simulink model "ROPOD_4Wheel_TdistZMPC_cntr"  (R2017b)
settings: Solver=FixedStepAuto  StartTime=0.0  StopTime=Inf  FixedStep=Ts  RelTol=1e-3
PreLoadFcn:
  | cd /home/robocup/RoPod/Force_dist_ZMPC_ROS
  | init_model
InitFcn:
  | cd /home/robocup/RoPod/Force_dist_ZMPC_ROS
  | init_model
values from neighbouring files (symbols this model uses):
  b_cx = 36.5    [RoPod_parameters.mat]
  b_cy = 36.5    [RoPod_parameters.mat]
  Fd_max = 70    [RoPod_parameters.mat]
  Fd_min = 20    [RoPod_parameters.mat]
  FFtheta_intia = 0    [init_model.m]
  FFxy_mass = 80    [init_model.m]
  Fr_max = 100    [RoPod_parameters.mat]
  Fr_min = -100    [RoPod_parameters.mat]
  k_cx = 1713    [RoPod_parameters.mat]
  k_cy = 4489    [RoPod_parameters.mat]
  max_hw_tau = 7.0    (= 7)    [init_model.m]
  Nwheels = 4    [init_model.m]
  pivot_offs_sws = [2.21 1.873 2.001 3.508]    [init_model.m]
  SW_COM1_ENABLE1 = hex2dec('0001')    [init_model.m]
  SW_COM1_ENABLE2 = hex2dec('0002')    [init_model.m]
  SW_COM1_MODE_TORQUE = bitshift(hex2dec('0000'),2)    [init_model.m]
  SW_COM1_MODE_VELOCITY = bitshift(hex2dec('0002'),2)    [init_model.m]
  SW_COM1_USE_TS = hex2dec('8000')    [init_model.m]
  sw_tau_2_curr = 1/motor_physical_parameters.torqueconstant.value    [init_model.m]
  Taucompfactor = 2.0    (= 2)    [init_model.m]
  Tinit = 1*Tslot    [init_model.m]
  Ts = 0.001    [init_model.m]
  Ts_MPC = 0.001    [init_model.m]
  Tsp = 1    [init_model.m]
  xA = [1 -1 0 0 0 0 0.0206696424966 -0.0206696424966 0 0 0.0298227588181 -0.0298227588181 ... (4080 elements, 102x40)]    [ZMPCx_parameters.mat]
  xBd_dis = [1.12932348493e-06 0.000225071897401 0 0]    [ZMPCx_parameters.mat]
  xF = [0 0 0 0 0 0 0 0 0 0 0 0 ... (80 elements, 20x4)]    [ZMPCx_parameters.mat]
  xH = [20 0 0 0 0 0 0 0 0 0 0 0 ... (1600 elements, 40x40)]    [ZMPCx_parameters.mat]
  xPhi = [0.995143909015 -0.967809158823 0 0 0.980727027327 -1.91066813489 0 0 0.957042868744 -2.81984596436 0 0 ... (320 elements, 80x4)]    [ZMPCx_parameters.mat]
  xrho = 144000    [ZMPCx_parameters.mat]
  xW = [0 0 -4300 4300 0 0 -4211.12053726 4211.12053726 0 0 -4082.88267435 4082.88267435 ... (328 elements, 82x4)]    [ZMPCx_parameters.mat]
  yA = [1 -1 0 0 0 0 0.0146537039222 -0.0146537039222 0 0 0.0255124036215 -0.0255124036215 ... (4080 elements, 102x40)]    [ZMPCy_parameters.mat]
  yBd_dis = [1.24492522358e-06 0.000248362591603 0 0]    [ZMPCy_parameters.mat]
  yF = [0.00191047141222 0.00156448969707 0.00119761396088 0.000813779538874 0.00041715000072 1.20724055612e-05 -0.00039696993291 -0.000805406662726 -0.00120863105559 -0.00160205155743 -0.00198114365531 -0.00234150147928 ... (80 elements, 20x4)]    [ZMPCy_parameters.mat]
  yH = [2.00000002801 0 2.31602594113e-08 0 1.80085634996e-08 0 1.26053094289e-08 0 7.00898668547e-09 0 1.2808124932e-09 0 ... (1600 elements, 40x40)]    [ZMPCy_parameters.mat]
  yPhi = [0.994411530671 -1.11489967371 0 0 0.977778317439 -2.20691845877 0 0 0.950389393786 -3.2640842851 0 0 ... (320 elements, 80x4)]    [ZMPCy_parameters.mat]
  yrho = 10000    [ZMPCy_parameters.mat]
  yW = [0 0 -4489 4489 0 0 -4423.21952309 4423.21952309 0 0 -4308.69434324 4308.69434324 ... (328 elements, 82x4)]    [ZMPCy_parameters.mat]
undefined symbols (not defined in the file or in its folder): DiscIntNeverNeededParam, Pose, ropod_kinmodel_param, Twist, Wrench
libraries: cstblocks x85, robotlib x60, simulink x41, SOEM_EtherCAT_Lib x5, robotcorelib x1
(part 3 of 6)

== system ROPOD_4Wheel_TdistZMPC_cntr/Non-ROS Ropod Controller/velocity_setpoint/Acceleration and Velocity Limits ==
  dq_setp : Inport
  base_conf : Inport  Port=2
  Bus Selector1 : BusSelector  OutputSignals=max_acc_xy,max_vel_xy
  Bus Selector2 : BusSelector  OutputSignals=max_acc_xy,max_vel_xy
  Bus Selector3 : BusSelector  OutputSignals=max_acc_theta,max_vel_theta
  Demux : Demux  Outputs=3
  Gain{,1..5} (6 alike) : Gain  Gain=-1
  Mux : Mux  Inputs=3
  Rate Limiter Dynamic : simulink/Discontinuities/Rate Limiter Dynamic
      settings: SourceProductName=Simulink
  Rate Limiter Dynamic1 : simulink/Discontinuities/Rate Limiter Dynamic
      settings: SourceProductName=Simulink
  Rate Limiter Dynamic2 : simulink/Discontinuities/Rate Limiter Dynamic
      settings: SourceProductName=Simulink
  Saturation Dynamic : simulink/Discontinuities/Saturation Dynamic  OutMin=[]  OutMax=[]  OutDataTypeStr=Inherit: Same as second input  OutDataType=fixdt(1, 16)  OutScaling=2^-10  DoSatur=off
  Saturation Dynamic1 : simulink/Discontinuities/Saturation Dynamic  OutMin=[]  OutMax=[]  OutDataTypeStr=Inherit: Same as second input  OutDataType=fixdt(1, 16)  OutScaling=2^-10  DoSatur=off
  Saturation Dynamic2 : simulink/Discontinuities/Saturation Dynamic  OutMin=[]  OutMax=[]  OutDataTypeStr=Inherit: Same as second input  OutDataType=fixdt(1, 16)  OutScaling=2^-10  DoSatur=off
  dq_loc : Outport
  wires:
  dq_setp/1 -> Demux/1
  Gain/1 -> Rate Limiter Dynamic/3
  Demux/1 -> Saturation Dynamic/2
  Gain1/1 -> Saturation Dynamic/3
  Saturation Dynamic/1 -> Rate Limiter Dynamic/2
  Demux/2 -> Saturation Dynamic1/2
  Gain3/1 -> Saturation Dynamic1/3
  Gain2/1 -> Rate Limiter Dynamic1/3
  Saturation Dynamic1/1 -> Rate Limiter Dynamic1/2
  Bus Selector2/1 -> Rate Limiter Dynamic1/1, Gain2/1  "<max_acc_xy>"
  Bus Selector2/2 -> Saturation Dynamic1/1, Gain3/1  "<max_vel_xy>"
  Bus Selector3/1 -> Rate Limiter Dynamic2/1, Gain4/1  "<max_acc_theta>"
  Saturation Dynamic2/1 -> Rate Limiter Dynamic2/2
  base_conf/1 -> Bus Selector3/1, Bus Selector2/1, Bus Selector1/1
  Demux/3 -> Saturation Dynamic2/2
  Gain5/1 -> Saturation Dynamic2/3
  Gain4/1 -> Rate Limiter Dynamic2/3
  Bus Selector3/2 -> Saturation Dynamic2/1, Gain5/1  "<max_vel_theta>"
  Mux/1 -> dq_loc/1
  Rate Limiter Dynamic/1 -> Mux/1
  Rate Limiter Dynamic1/1 -> Mux/2
  Rate Limiter Dynamic2/1 -> Mux/3
  Bus Selector1/2 -> Saturation Dynamic/1, Gain1/1  "<max_vel_xy>"
  Bus Selector1/1 -> Rate Limiter Dynamic/1, Gain/1  "<max_acc_xy>"

== system ROPOD_4Wheel_TdistZMPC_cntr/Non-ROS Ropod Controller/velocity_setpoint/Acceleration and Velocity Limits1 ==
  note: set 0 for testing
  note: if no vel commands are received after 0.5 sec, stop
  new_cmd : Inport
  dq_setp : Inport  Port=2
  Compare To Constant : simulink/Logic and Bit Operations/Compare To Constant  relop=>=  const=0.5  OutDataTypeStr=boolean
  Constant : Constant  Value=0
  Constant1 : Constant  Value=0
  Constant2 : Constant  Value=0
  Demux : Demux  Outputs=3
  Digital Clock : DigitalClock  SampleTime=Ts
  Enabled Delay : Delay  DelayLength=1  ShowEnablePort=on  SampleTime=Ts
      settings: InputPortMap=u0,e6
  Gain6 : Gain
  Mux : Mux  Inputs=3
  Subtract : Sum  Inputs=+-
  Switch : Switch  Criteria=u2 > Threshold
  Switch1 : Switch  Criteria=u2 > Threshold
  Switch2 : Switch  Criteria=u2 > Threshold
  dq_loc : Outport
  wires:
  Demux/1 -> Switch/3
  dq_setp/1 -> Demux/1
  new_cmd/1 -> Enabled Delay/2
  Digital Clock/1 -> Enabled Delay/1, Subtract/1
  Enabled Delay/1 -> Subtract/2
  Subtract/1 -> Compare To Constant/1
  Constant/1 -> Switch/1
  Constant1/1 -> Switch1/1
  Demux/2 -> Switch1/3
  Constant2/1 -> Switch2/1
  Demux/3 -> Switch2/3
  Compare To Constant/1 -> Gain6/1
  Mux/1 -> dq_loc/1
  Gain6/1 -> Switch2/2, Switch1/2, Switch/2
  Switch/1 -> Mux/1
  Switch1/1 -> Mux/2
  Switch2/1 -> Mux/3

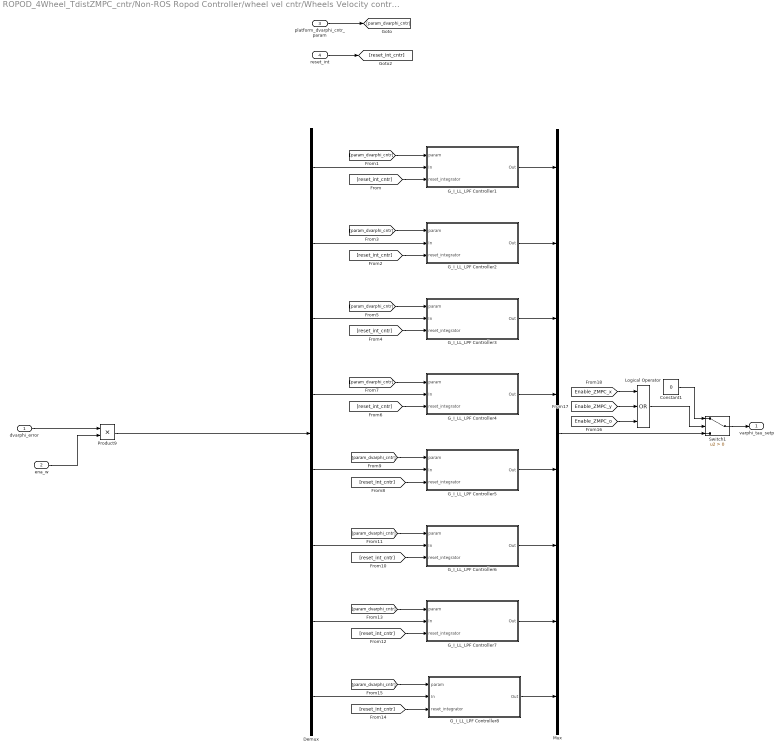
== system ROPOD_4Wheel_TdistZMPC_cntr/Non-ROS Ropod Controller/wheel vel cntr/Wheels Velocity controller ==
  dvarphi_error : Inport
  ena_w : Inport  Port=2
  platform_dvarphi_cntr_param : Inport  Port=3
  reset_int : Inport  Port=4
  Constant1 : Constant  Value=0
  Demux : Demux  Outputs=8
  G_I_LL_LPF Controller1 : Subsystem
  G_I_LL_LPF Controller2 : Subsystem
  G_I_LL_LPF Controller3 : Subsystem
  G_I_LL_LPF Controller4 : Subsystem
  G_I_LL_LPF Controller5 : Subsystem
  G_I_LL_LPF Controller6 : Subsystem
  G_I_LL_LPF Controller7 : Subsystem
  G_I_LL_LPF Controller8 : Subsystem
  Logical Operator : Logic  Operator=OR  Inputs=3  AllPortsSameDT=off  OutDataTypeStr=boolean
  Mux : Mux  Inputs=8
  Product9 : Product
  Switch1 : Switch  Criteria=u2 > Threshold
  varphi_tau_setp : Outport
  wires:
  ena_w/1 -> Product9/2
  Product9/1 -> Demux/1
  dvarphi_error/1 -> Product9/1
  [reset_int_cntr] -> G_I_LL_LPF Controller1/3(reset_integrator)
  Demux/1 -> G_I_LL_LPF Controller1/2(In)
  [param_dvarphi_cntr] -> G_I_LL_LPF Controller1/1(param)
  platform_dvarphi_cntr_param/1 -> [param_dvarphi_cntr]
  reset_int/1 -> [reset_int_cntr]
  [param_dvarphi_cntr] -> G_I_LL_LPF Controller2/1(param)
  [reset_int_cntr] -> G_I_LL_LPF Controller2/3(reset_integrator)
  Demux/2 -> G_I_LL_LPF Controller2/2(In)
  [reset_int_cntr] -> G_I_LL_LPF Controller4/3(reset_integrator)
  Demux/3 -> G_I_LL_LPF Controller3/2(In)
  Demux/4 -> G_I_LL_LPF Controller4/2(In)
  [param_dvarphi_cntr] -> G_I_LL_LPF Controller4/1(param)
  [param_dvarphi_cntr] -> G_I_LL_LPF Controller3/1(param)
  [reset_int_cntr] -> G_I_LL_LPF Controller3/3(reset_integrator)
  [param_dvarphi_cntr] -> G_I_LL_LPF Controller5/1(param)
  Demux/8 -> G_I_LL_LPF Controller8/2(In)
  [param_dvarphi_cntr] -> G_I_LL_LPF Controller7/1(param)
  [param_dvarphi_cntr] -> G_I_LL_LPF Controller8/1(param)
  [reset_int_cntr] -> G_I_LL_LPF Controller8/3(reset_integrator)
  [param_dvarphi_cntr] -> G_I_LL_LPF Controller6/1(param)
  [reset_int_cntr] -> G_I_LL_LPF Controller7/3(reset_integrator)
  Demux/6 -> G_I_LL_LPF Controller6/2(In)
  Demux/7 -> G_I_LL_LPF Controller7/2(In)
  [reset_int_cntr] -> G_I_LL_LPF Controller6/3(reset_integrator)
  [reset_int_cntr] -> G_I_LL_LPF Controller5/3(reset_integrator)
  Demux/5 -> G_I_LL_LPF Controller5/2(In)
  G_I_LL_LPF Controller1/1(Out) -> Mux/1
  G_I_LL_LPF Controller2/1(Out) -> Mux/2
  G_I_LL_LPF Controller4/1(Out) -> Mux/4
  G_I_LL_LPF Controller3/1(Out) -> Mux/3
  G_I_LL_LPF Controller5/1(Out) -> Mux/5
  G_I_LL_LPF Controller6/1(Out) -> Mux/6
  G_I_LL_LPF Controller7/1(Out) -> Mux/7
  G_I_LL_LPF Controller8/1(Out) -> Mux/8
  Constant1/1 -> Switch1/1
  Logical Operator/1 -> Switch1/2
  [Enable_ZMPC_y] -> Logical Operator/2
  [Enable_ZMPC_o] -> Logical Operator/3
  [Enable_ZMPC_x] -> Logical Operator/1
  Switch1/1 -> varphi_tau_setp/1
  Mux/1 -> Switch1/3

== system ROPOD_4Wheel_TdistZMPC_cntr/Non-ROS Ropod Controller/platform vel cntr/Bumper Interaction Controller/Angle controller ==
  angle : Inport
  Enable : EnablePort  StatesWhenEnabling=reset
  D : Gain
  Discrete-Time Integrator : DiscreteIntegrator  InitialConditionSetting=State (most efficient)  SampleTime=-1  ICPrevOutput=DiscIntNeverNeededParam  ICPrevScaledInput=DiscIntNeverNeededParam
  Discrete-Time Integrator1 : DiscreteIntegrator  InitialConditionSetting=State (most efficient)  SampleTime=-1  ICPrevOutput=DiscIntNeverNeededParam  ICPrevScaledInput=DiscIntNeverNeededParam
  I : Gain
  P : Gain  Gain=4000
  Ref_speed : Constant  Value=0
  Sum : Sum  Inputs=|+-
  Sum1 : Sum  Inputs=+|++
  Sum2 : Sum  Inputs=|+-
  u_N : Outport  OutputWhenDisabled=reset  InitialOutput=0
  wires:
  Sum1/1 -> u_N/1
  Discrete-Time Integrator/1 -> Sum1/1
  I/1 -> Discrete-Time Integrator/1
  angle/1 -> Sum2/2
  Sum2/1 -> P/1, D/1, I/1
  Ref_speed/1 -> Sum2/1
  Discrete-Time Integrator1/1 -> Sum/2
  Sum/1 -> Discrete-Time Integrator1/1, Sum1/3
  P/1 -> Sum1/2
  D/1 -> Sum/1

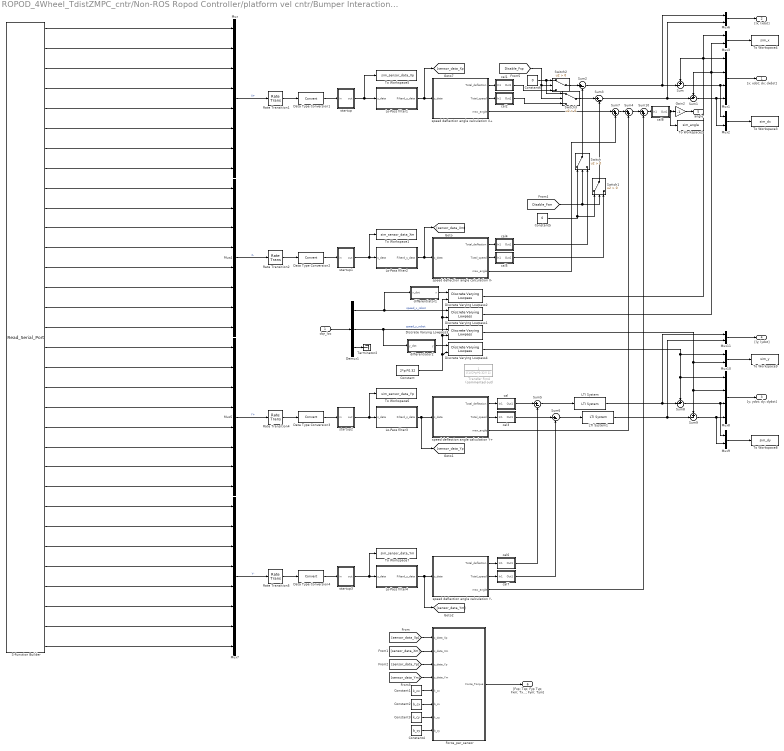
== system ROPOD_4Wheel_TdistZMPC_cntr/Non-ROS Ropod Controller/platform vel cntr/Bumper Interaction Controller/Bumper_system ==
  dqr_loc : Inport
  Constant : Constant  Value=2*pi*0.32
  Constant1 : Constant  Value=k_cx
  Constant2 : Constant  Value=b_cx
  Constant3 : Constant  Value=k_cy
  Constant4 : Constant  Value=b_cy
  Constant5 : Constant  Value=0
  Constant6 : Constant  Value=0
  Data Type Conversion{1..4} (4 alike) : DataTypeConversion
  Demux1 : Demux  Outputs=3
  Discrete Varying Lowpass{1..4} (4 alike) : cstblocks/Linear Parameter Varying/Discrete Varying Lowpass  N=1  w0=0  Ts=Ts
      settings: SourceProductName=Control System Toolbox  SourceProductBaseCode=CT
  Force_per_sensor : MATLAB Function  TreatAsAtomicUnit=on
  Gain2 : Gain  Gain=-1
  LTI System : cstblocks/LTI System  sys=hpfD_Bumper  IC=[]
  LTI System1 : cstblocks/LTI System  sys=hpfD_Bumper  IC=[]
  Lo-Pass filter1 : Subsystem
  Lo-Pass filter2 : Subsystem
  Lo-Pass filter3 : Subsystem
  Lo-Pass filter4 : Subsystem
  Mux{,4..5,7} (4 alike) : Mux  Inputs=8
  Mux1 : Mux
  Mux{2..3,6,9..11} (6 alike) : Mux  Inputs=2
  Mux8 : Mux
  Rate Transition{1..2,4..5} (4 alike) : RateTransition
  S-Function Builder : S-Function  InitFcn=try, set_param(gcb,'FunctionName','Read_Serial_Port'), end  FunctionName=Read_Serial_Port  SFunctionModules=Read_Serial_Port_wrapper  SFunctionDeploymentMode=off  EnableBusSupport=off  mask(S-Function Builder){}
      mask help: Simulink:masks:SFunctionBuilder_MD
      mask init:
      | val = [[.9  0.75 0.75 1 1 .9 .9 1]',[1 1 0.75 0.75 .9 .9 1 .9]'];try , sys = get_param(gcb,'SfunBuilderFcnName');if isempty(sys), sys = get_param(gcb,'FunctionName'); end,catch, sys = get_param(gcb,'FunctionName'); end
      settings: CopyFcn=set_param(gcbh,'LinkStatus','none')  PreSaveFcn=try, set_param(gcb,'FunctionName','Read_Serial_Port'), end  OpenFcn=sfunctionwizard(gcbh)
      mask Display: plot(val(:,1),val(:,2)),disp(sys), port_label('output',1,'dxp1'), port_label('output',2,'dxp2'), port_label('output',3,'dxp3'), port_label('output',4,'dxp4'), port_label('output',5,'sxp1'), port_label('output',6,'sxp2'), port_label('output',7,'sxp3'), port_label('output',8,'sxp4'), port_label('output',9,'dxm1'), port_label('output',10,'dxm2'), port_label('output',11,'dxm3'), port_label('output',12,'dxm4'), port_label('output',13,'sxm1'), port_label('output',14,'sxm2'), port_label('output',15,'sxm3'), port_label('output',16,'sxm4'), port_label('output',17,'dyp1'), port_label('output',18,'dyp2'), port_label('output',19,'dyp3'), port_label('output',20,'dyp4'), port_label('output',21,'syp1'), port_label('output',22,'syp2'), port_label('output',23,'syp3'), port_label('output',24,'syp4'), port_label('output',25,'dym1'), port_label('output',26,'dym2'), port_label('output',27,'dym3'), port_label('output',28,'dym4'), port_label('output',29,'sym1'), port_label('output',30,'sym2'), port_label('output',31,'sym3'), port_label('output',32,'sym4')
  Sum{,1,8..9} (4 alike) : Sum  Inputs=+-|
  Sum10 : Sum  Inputs=|++
  Sum{2..3,5..6} (4 alike) : Sum  Inputs=|+-
  Sum4 : Sum  Inputs=|++
  Sum7 : Sum  Inputs=|++
  Switch{,1..3} (4 alike) : Switch  Criteria=u2 > Threshold
  Terminator2 : Terminator
  To Workspace1 : ToWorkspace  VariableName=sim_sensor_data_Xm  SampleTime=-1
      settings: Save2DSignal=2-D array (concatenate along first dimension)
  To Workspace2 : ToWorkspace  VariableName=sim_angle  SampleTime=-1
      settings: Save2DSignal=2-D array (concatenate along first dimension)
  To Workspace3 : ToWorkspace  VariableName=sim_dx  SampleTime=-1
      settings: Save2DSignal=2-D array (concatenate along first dimension)
  To Workspace4 : ToWorkspace  VariableName=sim_x  SampleTime=-1
      settings: Save2DSignal=2-D array (concatenate along first dimension)
  To Workspace5 : ToWorkspace  VariableName=sim_sensor_data_Xp  SampleTime=-1
      settings: Save2DSignal=2-D array (concatenate along first dimension)
  To Workspace6 : ToWorkspace  VariableName=sim_sensor_data_Yp  SampleTime=-1
      settings: Save2DSignal=2-D array (concatenate along first dimension)
  To Workspace7 : ToWorkspace  VariableName=sim_sensor_data_Ym  SampleTime=-1
      settings: Save2DSignal=2-D array (concatenate along first dimension)
  To Workspace8 : ToWorkspace  VariableName=sim_dy  SampleTime=-1
      settings: Save2DSignal=2-D array (concatenate along first dimension)
  To Workspace9 : ToWorkspace  VariableName=sim_y  SampleTime=-1
      settings: Save2DSignal=2-D array (concatenate along first dimension)
  Transfer Fcn4 : TransferFcn  Commented=on  Denominator=[(1/(2*pi*0.32)) 1]
  cal : Subsystem
  cal1 : Subsystem
  cal2 : Subsystem
  cal3 : Subsystem
  cal4 : Subsystem
  cal5 : Subsystem
  cal6 : Subsystem
  cal7 : Subsystem
  cal8 : Subsystem
  differentiator1 : Subsystem
  differentiator2 : Subsystem
  speed deflection angle calculation X+ : MATLAB Function  TreatAsAtomicUnit=on
  speed deflection angle calculation X- : MATLAB Function  TreatAsAtomicUnit=on
  speed deflection angle calculation Y+ : MATLAB Function  TreatAsAtomicUnit=on
  speed deflection angle calculation Y- : MATLAB Function  TreatAsAtomicUnit=on
  startup : Subsystem
  startup1 : Subsystem
  startup2 : Subsystem
  startup3 : Subsystem
  "[x; xdot; dx; dxdot]" : Outport
  "[lx; lxdot]" : Outport  Port=2
  "[y; ydot; dy; dydot]" : Outport  Port=3
  "[ly; lydot]" : Outport  Port=4
  angle : Outport  Port=5
  "[Fxp; Txp; Fyp Typ; Fxm; Txm; Fym; Tym] " : Outport  Port=6
  wires:
  Mux2/1 -> To Workspace3/1
  Mux6/1 -> "[lx; lxdot]"/1
  Mux1/1 -> "[x; xdot; dx; dxdot]"/1
  Sum/1 -> Mux2/1, Mux1/3
  Discrete Varying Lowpass2/1 -> Mux3/1, Mux1/1, Sum/1
  Sum1/1 -> Mux2/2, Mux1/4
  Discrete Varying Lowpass1/1 -> Mux3/2, Sum1/1, Mux1/2
  Mux3/1 -> To Workspace4/1
  Demux1/3 -> Terminator2/1
  Demux1/1 -> Discrete Varying Lowpass1/1, differentiator1/1(x_dot)  "speed_x_robot"
  dqr_loc/1 -> Demux1/1
  Demux1/2 -> Discrete Varying Lowpass3/1, differentiator2/1(y_dot)  "speed_y_robot"
  differentiator1/1(x) -> Discrete Varying Lowpass2/1
  Mux/1 -> Rate Transition1/1  "X+"
  Lo-Pass filter1/1(Filterd_s_data) -> [sensor_data_Xp], speed deflection angle calculation X+/1(s_data)
  Data Type Conversion1/1 -> startup/1(in)
  Rate Transition1/1 -> Data Type Conversion1/1
  Rate Transition2/1 -> Data Type Conversion2/1
  Data Type Conversion2/1 -> startup1/1(in)
  Mux4/1 -> Rate Transition2/1  "X-"
  Rate Transition4/1 -> Data Type Conversion3/1
  Data Type Conversion3/1 -> startup2/1(in)
  Lo-Pass filter3/1(Filterd_s_data) -> [sensor_data_Yp], speed deflection angle calculation Y+/1(s_data)
  Rate Transition5/1 -> Data Type Conversion4/1
  Data Type Conversion4/1 -> startup3/1(in)
  Lo-Pass filter4/1(Filterd_s_data) -> [sensor_data_Ym], speed deflection angle calculation Y-/1(s_data)
  Mux7/1 -> Rate Transition5/1  "Y-"
  Mux5/1 -> Rate Transition4/1  "Y+"
  speed deflection angle calculation X+/1(Total_deflection) -> cal1/1(In1)
  Switch/1 -> Sum2/2
  Switch1/1 -> Sum3/2
  speed deflection angle calculation X+/3(max_angle) -> Sum7/1
  speed deflection angle calculation Y-/3(max_angle) -> Sum10/2
  speed deflection angle calculation Y-/1(Total_deflection) -> cal6/1(In1)
  speed deflection angle calculation Y+/3(max_angle) -> Sum4/2
  speed deflection angle calculation Y+/2(Total_speed) -> cal3/1(In1)
  speed deflection angle calculation Y-/2(Total_speed) -> cal7/1(In1)
  Sum8/1 -> Mux9/1, Mux8/3
  Mux10/1 -> To Workspace9/1
  Mux8/1 -> "[y; ydot; dy; dydot]"/1
  Discrete Varying Lowpass4/1 -> Mux8/1, Sum8/1, Mux10/1
  Mux11/1 -> "[ly; lydot]"/1
  Sum9/1 -> Mux9/2, Mux8/4
  Mux9/1 -> To Workspace8/1
  Discrete Varying Lowpass3/1 -> Mux8/2, Sum9/1, Mux10/2
  differentiator2/1(y) -> Discrete Varying Lowpass4/1
  speed deflection angle calculation X-/3(max_angle) -> Sum7/2
  Sum7/1 -> Sum4/1
  Sum4/1 -> Sum10/1
  Sum10/1 -> cal8/1(In1)
  Sum5/1 -> LTI System/1
  Sum2/1 -> Sum/2, Mux6/1
  Sum3/1 -> Sum1/2, Mux6/2
  Sum6/1 -> LTI System1/1
  startup/1(out) -> To Workspace5/1, Lo-Pass filter1/1(s_data)
  startup1/1(out) -> Lo-Pass filter2/1(s_data), To Workspace1/1
  startup2/1(out) -> Lo-Pass filter3/1(s_data), To Workspace6/1
  startup3/1(out) -> Lo-Pass filter4/1(s_data), To Workspace7/1
  Constant/1 -> Discrete Varying Lowpass4/2, Discrete Varying Lowpass3/2, Discrete Varying Lowpass1/2, Discrete Varying Lowpass2/2
  S-Function Builder/26 -> Mux7/2
  S-Function Builder/31 -> Mux7/7
  S-Function Builder/20 -> Mux5/4
  S-Function Builder/18 -> Mux5/2
  S-Function Builder/25 -> Mux7/1
  S-Function Builder/13 -> Mux4/5
  S-Function Builder/23 -> Mux5/7
  S-Function Builder/15 -> Mux4/7
  S-Function Builder/22 -> Mux5/6
  S-Function Builder/14 -> Mux4/6
  S-Function Builder/17 -> Mux5/1
  S-Function Builder/32 -> Mux7/8
  S-Function Builder/7 -> Mux/7
  S-Function Builder/19 -> Mux5/3
  S-Function Builder/21 -> Mux5/5
  S-Function Builder/8 -> Mux/8
  S-Function Builder/5 -> Mux/5
  S-Function Builder/4 -> Mux/4
  S-Function Builder/29 -> Mux7/5
  S-Function Builder/6 -> Mux/6
  S-Function Builder/1 -> Mux/1
  S-Function Builder/3 -> Mux/3
  S-Function Builder/10 -> Mux4/2
  S-Function Builder/11 -> Mux4/3
  S-Function Builder/12 -> Mux4/4
  S-Function Builder/16 -> Mux4/8
  S-Function Builder/28 -> Mux7/4
  S-Function Builder/27 -> Mux7/3
  S-Function Builder/9 -> Mux4/1
  S-Function Builder/30 -> Mux7/6
  S-Function Builder/2 -> Mux/2
  S-Function Builder/24 -> Mux5/8
  [sensor_data_Xp] -> Force_per_sensor/1(s_data_Xp)
  [sensor_data_Xm] -> Force_per_sensor/2(s_data_Xm)
  [sensor_data_Yp] -> Force_per_sensor/3(s_data_Yp)
  [sensor_data_Ym] -> Force_per_sensor/4(s_data_Ym)
  Force_per_sensor/1(Force_Torque) -> "[Fxp; Txp; Fyp Typ; Fxm; Txm; Fym; Tym] "/1
  Constant1/1 -> Force_per_sensor/5(k_cx)
  Constant2/1 -> Force_per_sensor/6(b_cx)
  Constant3/1 -> Force_per_sensor/7(k_cy)
  Constant4/1 -> Force_per_sensor/8(b_cy)
  cal1/1(Out1) -> Switch2/3
  speed deflection angle calculation X+/2(Total_speed) -> cal2/1(In1)
  cal2/1(Out1) -> Switch3/3
  speed deflection angle calculation X-/1(Total_deflection) -> cal4/1(In1)
  speed deflection angle calculation X-/2(Total_speed) -> cal5/1(In1)
  speed deflection angle calculation Y+/1(Total_deflection) -> cal/1(In1)
  cal/1(Out1) -> Sum5/1
  cal3/1(Out1) -> Sum6/1
  cal6/1(Out1) -> Sum5/2
  cal7/1(Out1) -> Sum6/2
  [Disable_Fxm] -> Switch/2, Switch1/2
  cal4/1(Out1) -> Switch/3
  cal5/1(Out1) -> Switch1/3
  Constant5/1 -> Switch1/1, Switch/1
  Switch2/1 -> Sum2/1
  Switch3/1 -> Sum3/1
  Constant6/1 -> Switch3/1, Switch2/1
  [Disable_Fxp] -> Switch2/2, Switch3/2
  LTI System/1 -> Sum8/2, Mux11/1
  LTI System1/1 -> Sum9/2, Mux11/2
  Lo-Pass filter2/1(Filterd_s_data) -> [sensor_data_Xm], speed deflection angle calculation X-/1(s_data)
  cal8/1(Out1) -> To Workspace2/1, Gain2/1
  Gain2/1 -> angle/1

== system ROPOD_4Wheel_TdistZMPC_cntr/Non-ROS Ropod Controller/platform vel cntr/Bumper Interaction Controller/ZMPC_x ==
  "[x; xdot; d; ddot]" : Inport
  Fd_min : Inport  Port=2
  Fd_max : Inport  Port=3
  Enable : EnablePort  StatesWhenEnabling=reset
  Constant1 : Constant  Value=xPhi
  Constant16 : Constant  Value=xH
  Constant2 : Constant  Value=xBd_dis
  Constant26 : Constant  Value=Fr_min
  Constant27 : Constant  Value=Fr_max
  Constant28 : Constant  Value=xF
  Constant30 : Constant  Value=xA
  Constant31 : Constant  Value=xW
  Constant32 : Constant  Value=xrho
  Delay{,1..4} (5 alike) : Delay  DelayLength=1  SampleTime=Ts_MPC
  Delay6 : Delay  DelayLength=1  InitialCondition=10  SampleTime=Ts_MPC
  To Workspace10 : ToWorkspace  VariableName=sim_x_e  SampleTime=-1
      settings: Save2DSignal=2-D array (concatenate along first dimension)
  To Workspace9 : ToWorkspace  VariableName=sim_x_uf  SampleTime=-1
      settings: Save2DSignal=2-D array (concatenate along first dimension)
  Zone MPC : MATLAB Function  TreatAsAtomicUnit=on  SystemSampleTime=Ts_MPC
  Fx : Outport  OutputWhenDisabled=reset  InitialOutput=0
  Feasability : Outport  Port=2  OutputWhenDisabled=reset  InitialOutput=0
  wires:
  Constant27/1 -> Zone MPC/4(Fr_max)
  Zone MPC/4(exitflag) -> Feasability/1, Delay1/1
  Delay/1 -> Zone MPC/15(mv_old)
  Delay4/1 -> Zone MPC/13(epsilon_old)
  Constant31/1 -> Zone MPC/10(W)
  Constant16/1 -> Zone MPC/7(H)
  Constant28/1 -> Zone MPC/8(F)
  Zone MPC/5(iA) -> Delay2/1
  Fd_max/1 -> Zone MPC/2(Fd_max)
  Constant26/1 -> Zone MPC/5(Fr_min)
  Delay3/1 -> Zone MPC/14(uf_old)
  Fd_min/1 -> Zone MPC/3(Fd_min)
  Constant1/1 -> Zone MPC/11(Phi)
  Zone MPC/6(s) -> Delay6/1
  Delay6/1 -> Zone MPC/18(s_old)
  Zone MPC/1(epsilon) -> To Workspace10/1, Delay4/1
  Zone MPC/2(u_f) -> To Workspace9/1, Delay3/1
  Constant32/1 -> Zone MPC/12(rho)
  Constant30/1 -> Zone MPC/9(A)
  Delay1/1 -> Zone MPC/16(exitflag_old)
  Delay2/1 -> Zone MPC/17(iA0)
  Constant2/1 -> Zone MPC/6(Bd_dis)
  "[x; xdot; d; ddot]"/1 -> Zone MPC/1(mo)
  Zone MPC/3(mv) -> Delay/1, Fx/1

== system ROPOD_4Wheel_TdistZMPC_cntr/Non-ROS Ropod Controller/platform vel cntr/Bumper Interaction Controller/ZMPC_y ==
  "[x; xdot; d; ddot]" : Inport
  Fd_min : Inport  Port=2
  Fd_max : Inport  Port=3
  Enable : EnablePort  StatesWhenEnabling=reset
  Constant1 : Constant  Value=yPhi
  Constant16 : Constant  Value=yH
  Constant2 : Constant  Value=yBd_dis
  Constant26 : Constant  Value=Fr_min
  Constant27 : Constant  Value=Fr_max
  Constant28 : Constant  Value=yF
  Constant30 : Constant  Value=yA
  Constant31 : Constant  Value=yW
  Constant32 : Constant  Value=yrho
  Delay{,1..4} (5 alike) : Delay  DelayLength=1  SampleTime=Ts_MPC
  Delay6 : Delay  DelayLength=1  InitialCondition=10  SampleTime=Ts_MPC
  To Workspace10 : ToWorkspace  VariableName=sim_y_e  SampleTime=-1
      settings: Save2DSignal=2-D array (concatenate along first dimension)
  To Workspace9 : ToWorkspace  VariableName=sim_y_uf  SampleTime=-1
      settings: Save2DSignal=2-D array (concatenate along first dimension)
  Zone MPC : MATLAB Function  TreatAsAtomicUnit=on  SystemSampleTime=Ts_MPC
  Fx : Outport  OutputWhenDisabled=reset  InitialOutput=0
  Feasability : Outport  Port=2  OutputWhenDisabled=reset  InitialOutput=0
  wires:
  Zone MPC/3(mv) -> Fx/1, Delay/1
  "[x; xdot; d; ddot]"/1 -> Zone MPC/1(mo)
  Constant2/1 -> Zone MPC/6(Bd_dis)
  Delay2/1 -> Zone MPC/17(iA0)
  Delay1/1 -> Zone MPC/16(exitflag_old)
  Constant30/1 -> Zone MPC/9(A)
  Constant32/1 -> Zone MPC/12(rho)
  Zone MPC/2(u_f) -> Delay3/1, To Workspace9/1
  Zone MPC/1(epsilon) -> Delay4/1, To Workspace10/1
  Delay6/1 -> Zone MPC/18(s_old)
  Zone MPC/6(s) -> Delay6/1
  Constant1/1 -> Zone MPC/11(Phi)
  Fd_min/1 -> Zone MPC/3(Fd_min)
  Delay3/1 -> Zone MPC/14(uf_old)
  Constant26/1 -> Zone MPC/5(Fr_min)
  Fd_max/1 -> Zone MPC/2(Fd_max)
  Zone MPC/5(iA) -> Delay2/1
  Constant28/1 -> Zone MPC/8(F)
  Constant16/1 -> Zone MPC/7(H)
  Constant31/1 -> Zone MPC/10(W)
  Delay4/1 -> Zone MPC/13(epsilon_old)
  Delay/1 -> Zone MPC/15(mv_old)
  Zone MPC/4(exitflag) -> Delay1/1, Feasability/1
  Constant27/1 -> Zone MPC/4(Fr_max)

== system ROPOD_4Wheel_TdistZMPC_cntr/Non-ROS Ropod Controller/platform vel cntr/Platorm Velocity controller/G_I_LL_LPF Controller1 ==
  param : Inport
  In : Inport  Port=2
  reset_integrator : Inport  Port=3
  Bus Selector : BusSelector  OutputSignals=P_gain,I_freq_hz,LL_zero_fhz,LL_pole_fhz,LPF_fhz
  Discrete Varying Lowpass3 : cstblocks/Linear Parameter Varying/Discrete Varying Lowpass  N=1  w0=0  Ts=Ts
      settings: SourceProductName=Control System Toolbox  SourceProductBaseCode=CT
  Gain2 : Gain  Gain=2*pi
  Product5 : Product
  Shapeit Integrator (Tustin) : Subsystem
  Shapeit Lead-Lag (Tustin) : Subsystem
  Out : Outport
  wires:
  Gain2/1 -> Discrete Varying Lowpass3/2
  Product5/1 -> Shapeit Integrator (Tustin)/1(In)
  Discrete Varying Lowpass3/1 -> Out/1
  Shapeit Integrator (Tustin)/1(Out) -> Shapeit Lead-Lag (Tustin)/1(In)
  Bus Selector/1 -> Product5/2  "<P_gain>"
  Bus Selector/2 -> Shapeit Integrator (Tustin)/2(I_fhz)  "<I_freq_hz>"
  param/1 -> Bus Selector/1
  Bus Selector/5 -> Gain2/1  "<LPF_fhz>"
  Bus Selector/4 -> Shapeit Lead-Lag (Tustin)/3(fp)  "<LL_pole_fhz>"
  reset_integrator/1 -> Shapeit Integrator (Tustin)/3(reset)
  Bus Selector/3 -> Shapeit Lead-Lag (Tustin)/2(fz)  "<LL_zero_fhz>"
  Shapeit Lead-Lag (Tustin)/1(Out) -> Discrete Varying Lowpass3/1
  In/1 -> Product5/1

== system ROPOD_4Wheel_TdistZMPC_cntr/Non-ROS Ropod Controller/platform vel cntr/Platorm Velocity controller/G_I_LL_LPF Controller2 ==
  param : Inport
  In : Inport  Port=2
  reset_integrator : Inport  Port=3
  Bus Selector : BusSelector  OutputSignals=P_gain,I_freq_hz,LL_zero_fhz,LL_pole_fhz,LPF_fhz
  Discrete Varying Lowpass3 : cstblocks/Linear Parameter Varying/Discrete Varying Lowpass  N=1  w0=0  Ts=Ts
      settings: SourceProductName=Control System Toolbox  SourceProductBaseCode=CT
  Gain2 : Gain  Gain=2*pi
  Product5 : Product
  Shapeit Integrator (Tustin) : Subsystem
  Shapeit Lead-Lag (Tustin) : Subsystem
  Out : Outport
  wires:
  Gain2/1 -> Discrete Varying Lowpass3/2
  Product5/1 -> Shapeit Integrator (Tustin)/1(In)
  Discrete Varying Lowpass3/1 -> Out/1
  Shapeit Integrator (Tustin)/1(Out) -> Shapeit Lead-Lag (Tustin)/1(In)
  Bus Selector/1 -> Product5/2  "<P_gain>"
  Bus Selector/2 -> Shapeit Integrator (Tustin)/2(I_fhz)  "<I_freq_hz>"
  param/1 -> Bus Selector/1
  Bus Selector/5 -> Gain2/1  "<LPF_fhz>"
  Bus Selector/4 -> Shapeit Lead-Lag (Tustin)/3(fp)  "<LL_pole_fhz>"
  reset_integrator/1 -> Shapeit Integrator (Tustin)/3(reset)
  Bus Selector/3 -> Shapeit Lead-Lag (Tustin)/2(fz)  "<LL_zero_fhz>"
  Shapeit Lead-Lag (Tustin)/1(Out) -> Discrete Varying Lowpass3/1
  In/1 -> Product5/1

== system ROPOD_4Wheel_TdistZMPC_cntr/Non-ROS Ropod Controller/platform vel cntr/Platorm Velocity controller/G_I_LL_LPF Controller3 ==
  param : Inport
  In : Inport  Port=2
  reset_integrator : Inport  Port=3
  Bus Selector : BusSelector  OutputSignals=P_gain,I_freq_hz,LL_zero_fhz,LL_pole_fhz,LPF_fhz
  Discrete Varying Lowpass3 : cstblocks/Linear Parameter Varying/Discrete Varying Lowpass  N=1  w0=0  Ts=Ts
      settings: SourceProductName=Control System Toolbox  SourceProductBaseCode=CT
  Gain2 : Gain  Gain=2*pi
  Product5 : Product
  Shapeit Integrator (Tustin) : Subsystem
  Shapeit Lead-Lag (Tustin) : Subsystem
  Out : Outport
  wires:
  Gain2/1 -> Discrete Varying Lowpass3/2
  Product5/1 -> Shapeit Integrator (Tustin)/1(In)
  Discrete Varying Lowpass3/1 -> Out/1
  Shapeit Integrator (Tustin)/1(Out) -> Shapeit Lead-Lag (Tustin)/1(In)
  Bus Selector/1 -> Product5/2  "<P_gain>"
  Bus Selector/2 -> Shapeit Integrator (Tustin)/2(I_fhz)  "<I_freq_hz>"
  param/1 -> Bus Selector/1
  Bus Selector/5 -> Gain2/1  "<LPF_fhz>"
  Bus Selector/4 -> Shapeit Lead-Lag (Tustin)/3(fp)  "<LL_pole_fhz>"
  reset_integrator/1 -> Shapeit Integrator (Tustin)/3(reset)
  Bus Selector/3 -> Shapeit Lead-Lag (Tustin)/2(fz)  "<LL_zero_fhz>"
  Shapeit Lead-Lag (Tustin)/1(Out) -> Discrete Varying Lowpass3/1
  In/1 -> Product5/1

== system ROPOD_4Wheel_TdistZMPC_cntr/Non-ROS Ropod Controller/wheel vel cntr/Wheels Velocity controller/G_I_LL_LPF Controller1 ==
  param : Inport
  In : Inport  Port=2
  reset_integrator : Inport  Port=3
  Bus Selector : BusSelector  OutputSignals=P_gain,I_freq_hz,LL_zero_fhz,LL_pole_fhz,LPF_fhz
  Discrete Varying Lowpass3 : cstblocks/Linear Parameter Varying/Discrete Varying Lowpass  N=1  w0=0  Ts=Ts
      settings: SourceProductName=Control System Toolbox  SourceProductBaseCode=CT
  Gain2 : Gain  Gain=2*pi
  Product5 : Product
  Shapeit Integrator (Tustin) : Subsystem
  Shapeit Lead-Lag (Tustin) : Subsystem
  Out : Outport
  wires:
  Gain2/1 -> Discrete Varying Lowpass3/2
  Product5/1 -> Shapeit Integrator (Tustin)/1(In)
  Discrete Varying Lowpass3/1 -> Out/1
  Shapeit Integrator (Tustin)/1(Out) -> Shapeit Lead-Lag (Tustin)/1(In)
  Bus Selector/1 -> Product5/2  "<P_gain>"
  Bus Selector/2 -> Shapeit Integrator (Tustin)/2(I_fhz)  "<I_freq_hz>"
  param/1 -> Bus Selector/1
  Bus Selector/5 -> Gain2/1  "<LPF_fhz>"
  Bus Selector/4 -> Shapeit Lead-Lag (Tustin)/3(fp)  "<LL_pole_fhz>"
  reset_integrator/1 -> Shapeit Integrator (Tustin)/3(reset)
  Bus Selector/3 -> Shapeit Lead-Lag (Tustin)/2(fz)  "<LL_zero_fhz>"
  Shapeit Lead-Lag (Tustin)/1(Out) -> Discrete Varying Lowpass3/1
  In/1 -> Product5/1

== system ROPOD_4Wheel_TdistZMPC_cntr/Non-ROS Ropod Controller/wheel vel cntr/Wheels Velocity controller/G_I_LL_LPF Controller2 ==
  param : Inport
  In : Inport  Port=2
  reset_integrator : Inport  Port=3
  Bus Selector : BusSelector  OutputSignals=P_gain,I_freq_hz,LL_zero_fhz,LL_pole_fhz,LPF_fhz
  Discrete Varying Lowpass3 : cstblocks/Linear Parameter Varying/Discrete Varying Lowpass  N=1  w0=0  Ts=Ts
      settings: SourceProductName=Control System Toolbox  SourceProductBaseCode=CT
  Gain2 : Gain  Gain=2*pi
  Product5 : Product
  Shapeit Integrator (Tustin) : Subsystem
  Shapeit Lead-Lag (Tustin) : Subsystem
  Out : Outport
  wires:
  Gain2/1 -> Discrete Varying Lowpass3/2
  Product5/1 -> Shapeit Integrator (Tustin)/1(In)
  Discrete Varying Lowpass3/1 -> Out/1
  Shapeit Integrator (Tustin)/1(Out) -> Shapeit Lead-Lag (Tustin)/1(In)
  Bus Selector/1 -> Product5/2  "<P_gain>"
  Bus Selector/2 -> Shapeit Integrator (Tustin)/2(I_fhz)  "<I_freq_hz>"
  param/1 -> Bus Selector/1
  Bus Selector/5 -> Gain2/1  "<LPF_fhz>"
  Bus Selector/4 -> Shapeit Lead-Lag (Tustin)/3(fp)  "<LL_pole_fhz>"
  reset_integrator/1 -> Shapeit Integrator (Tustin)/3(reset)
  Bus Selector/3 -> Shapeit Lead-Lag (Tustin)/2(fz)  "<LL_zero_fhz>"
  Shapeit Lead-Lag (Tustin)/1(Out) -> Discrete Varying Lowpass3/1
  In/1 -> Product5/1

== system ROPOD_4Wheel_TdistZMPC_cntr/Non-ROS Ropod Controller/wheel vel cntr/Wheels Velocity controller/G_I_LL_LPF Controller3 ==
  param : Inport
  In : Inport  Port=2
  reset_integrator : Inport  Port=3
  Bus Selector : BusSelector  OutputSignals=P_gain,I_freq_hz,LL_zero_fhz,LL_pole_fhz,LPF_fhz
  Discrete Varying Lowpass3 : cstblocks/Linear Parameter Varying/Discrete Varying Lowpass  N=1  w0=0  Ts=Ts
      settings: SourceProductName=Control System Toolbox  SourceProductBaseCode=CT
  Gain2 : Gain  Gain=2*pi
  Product5 : Product
  Shapeit Integrator (Tustin) : Subsystem
  Shapeit Lead-Lag (Tustin) : Subsystem
  Out : Outport
  wires:
  Gain2/1 -> Discrete Varying Lowpass3/2
  Product5/1 -> Shapeit Integrator (Tustin)/1(In)
  Discrete Varying Lowpass3/1 -> Out/1
  Shapeit Integrator (Tustin)/1(Out) -> Shapeit Lead-Lag (Tustin)/1(In)
  Bus Selector/1 -> Product5/2  "<P_gain>"
  Bus Selector/2 -> Shapeit Integrator (Tustin)/2(I_fhz)  "<I_freq_hz>"
  param/1 -> Bus Selector/1
  Bus Selector/5 -> Gain2/1  "<LPF_fhz>"
  Bus Selector/4 -> Shapeit Lead-Lag (Tustin)/3(fp)  "<LL_pole_fhz>"
  reset_integrator/1 -> Shapeit Integrator (Tustin)/3(reset)
  Bus Selector/3 -> Shapeit Lead-Lag (Tustin)/2(fz)  "<LL_zero_fhz>"
  Shapeit Lead-Lag (Tustin)/1(Out) -> Discrete Varying Lowpass3/1
  In/1 -> Product5/1

== system ROPOD_4Wheel_TdistZMPC_cntr/Non-ROS Ropod Controller/wheel vel cntr/Wheels Velocity controller/G_I_LL_LPF Controller4 ==
  param : Inport
  In : Inport  Port=2
  reset_integrator : Inport  Port=3
  Bus Selector : BusSelector  OutputSignals=P_gain,I_freq_hz,LL_zero_fhz,LL_pole_fhz,LPF_fhz
  Discrete Varying Lowpass3 : cstblocks/Linear Parameter Varying/Discrete Varying Lowpass  N=1  w0=0  Ts=Ts
      settings: SourceProductName=Control System Toolbox  SourceProductBaseCode=CT
  Gain2 : Gain  Gain=2*pi
  Product5 : Product
  Shapeit Integrator (Tustin) : Subsystem
  Shapeit Lead-Lag (Tustin) : Subsystem
  Out : Outport
  wires:
  Gain2/1 -> Discrete Varying Lowpass3/2
  Product5/1 -> Shapeit Integrator (Tustin)/1(In)
  Discrete Varying Lowpass3/1 -> Out/1
  Shapeit Integrator (Tustin)/1(Out) -> Shapeit Lead-Lag (Tustin)/1(In)
  Bus Selector/1 -> Product5/2  "<P_gain>"
  Bus Selector/2 -> Shapeit Integrator (Tustin)/2(I_fhz)  "<I_freq_hz>"
  param/1 -> Bus Selector/1
  Bus Selector/5 -> Gain2/1  "<LPF_fhz>"
  Bus Selector/4 -> Shapeit Lead-Lag (Tustin)/3(fp)  "<LL_pole_fhz>"
  reset_integrator/1 -> Shapeit Integrator (Tustin)/3(reset)
  Bus Selector/3 -> Shapeit Lead-Lag (Tustin)/2(fz)  "<LL_zero_fhz>"
  Shapeit Lead-Lag (Tustin)/1(Out) -> Discrete Varying Lowpass3/1
  In/1 -> Product5/1

== system ROPOD_4Wheel_TdistZMPC_cntr/Non-ROS Ropod Controller/wheel vel cntr/Wheels Velocity controller/G_I_LL_LPF Controller5 ==
  param : Inport
  In : Inport  Port=2
  reset_integrator : Inport  Port=3
  Bus Selector : BusSelector  OutputSignals=P_gain,I_freq_hz,LL_zero_fhz,LL_pole_fhz,LPF_fhz
  Discrete Varying Lowpass3 : cstblocks/Linear Parameter Varying/Discrete Varying Lowpass  N=1  w0=0  Ts=Ts
      settings: SourceProductName=Control System Toolbox  SourceProductBaseCode=CT
  Gain2 : Gain  Gain=2*pi
  Product5 : Product
  Shapeit Integrator (Tustin) : Subsystem
  Shapeit Lead-Lag (Tustin) : Subsystem
  Out : Outport
  wires:
  Gain2/1 -> Discrete Varying Lowpass3/2
  Product5/1 -> Shapeit Integrator (Tustin)/1(In)
  Discrete Varying Lowpass3/1 -> Out/1
  Shapeit Integrator (Tustin)/1(Out) -> Shapeit Lead-Lag (Tustin)/1(In)
  Bus Selector/1 -> Product5/2  "<P_gain>"
  Bus Selector/2 -> Shapeit Integrator (Tustin)/2(I_fhz)  "<I_freq_hz>"
  param/1 -> Bus Selector/1
  Bus Selector/5 -> Gain2/1  "<LPF_fhz>"
  Bus Selector/4 -> Shapeit Lead-Lag (Tustin)/3(fp)  "<LL_pole_fhz>"
  reset_integrator/1 -> Shapeit Integrator (Tustin)/3(reset)
  Bus Selector/3 -> Shapeit Lead-Lag (Tustin)/2(fz)  "<LL_zero_fhz>"
  Shapeit Lead-Lag (Tustin)/1(Out) -> Discrete Varying Lowpass3/1
  In/1 -> Product5/1

== system ROPOD_4Wheel_TdistZMPC_cntr/Non-ROS Ropod Controller/wheel vel cntr/Wheels Velocity controller/G_I_LL_LPF Controller6 ==
  param : Inport
  In : Inport  Port=2
  reset_integrator : Inport  Port=3
  Bus Selector : BusSelector  OutputSignals=P_gain,I_freq_hz,LL_zero_fhz,LL_pole_fhz,LPF_fhz
  Discrete Varying Lowpass3 : cstblocks/Linear Parameter Varying/Discrete Varying Lowpass  N=1  w0=0  Ts=Ts
      settings: SourceProductName=Control System Toolbox  SourceProductBaseCode=CT
  Gain2 : Gain  Gain=2*pi
  Product5 : Product
  Shapeit Integrator (Tustin) : Subsystem
  Shapeit Lead-Lag (Tustin) : Subsystem
  Out : Outport
  wires:
  Gain2/1 -> Discrete Varying Lowpass3/2
  Product5/1 -> Shapeit Integrator (Tustin)/1(In)
  Discrete Varying Lowpass3/1 -> Out/1
  Shapeit Integrator (Tustin)/1(Out) -> Shapeit Lead-Lag (Tustin)/1(In)
  Bus Selector/1 -> Product5/2  "<P_gain>"
  Bus Selector/2 -> Shapeit Integrator (Tustin)/2(I_fhz)  "<I_freq_hz>"
  param/1 -> Bus Selector/1
  Bus Selector/5 -> Gain2/1  "<LPF_fhz>"
  Bus Selector/4 -> Shapeit Lead-Lag (Tustin)/3(fp)  "<LL_pole_fhz>"
  reset_integrator/1 -> Shapeit Integrator (Tustin)/3(reset)
  Bus Selector/3 -> Shapeit Lead-Lag (Tustin)/2(fz)  "<LL_zero_fhz>"
  Shapeit Lead-Lag (Tustin)/1(Out) -> Discrete Varying Lowpass3/1
  In/1 -> Product5/1

== system ROPOD_4Wheel_TdistZMPC_cntr/Non-ROS Ropod Controller/wheel vel cntr/Wheels Velocity controller/G_I_LL_LPF Controller7 ==
  param : Inport
  In : Inport  Port=2
  reset_integrator : Inport  Port=3
  Bus Selector : BusSelector  OutputSignals=P_gain,I_freq_hz,LL_zero_fhz,LL_pole_fhz,LPF_fhz
  Discrete Varying Lowpass3 : cstblocks/Linear Parameter Varying/Discrete Varying Lowpass  N=1  w0=0  Ts=Ts
      settings: SourceProductName=Control System Toolbox  SourceProductBaseCode=CT
  Gain2 : Gain  Gain=2*pi
  Product5 : Product
  Shapeit Integrator (Tustin) : Subsystem
  Shapeit Lead-Lag (Tustin) : Subsystem
  Out : Outport
  wires:
  Gain2/1 -> Discrete Varying Lowpass3/2
  Product5/1 -> Shapeit Integrator (Tustin)/1(In)
  Discrete Varying Lowpass3/1 -> Out/1
  Shapeit Integrator (Tustin)/1(Out) -> Shapeit Lead-Lag (Tustin)/1(In)
  Bus Selector/1 -> Product5/2  "<P_gain>"
  Bus Selector/2 -> Shapeit Integrator (Tustin)/2(I_fhz)  "<I_freq_hz>"
  param/1 -> Bus Selector/1
  Bus Selector/5 -> Gain2/1  "<LPF_fhz>"
  Bus Selector/4 -> Shapeit Lead-Lag (Tustin)/3(fp)  "<LL_pole_fhz>"
  reset_integrator/1 -> Shapeit Integrator (Tustin)/3(reset)
  Bus Selector/3 -> Shapeit Lead-Lag (Tustin)/2(fz)  "<LL_zero_fhz>"
  Shapeit Lead-Lag (Tustin)/1(Out) -> Discrete Varying Lowpass3/1
  In/1 -> Product5/1

== system ROPOD_4Wheel_TdistZMPC_cntr/Non-ROS Ropod Controller/wheel vel cntr/Wheels Velocity controller/G_I_LL_LPF Controller8 ==
  param : Inport
  In : Inport  Port=2
  reset_integrator : Inport  Port=3
  Bus Selector : BusSelector  OutputSignals=P_gain,I_freq_hz,LL_zero_fhz,LL_pole_fhz,LPF_fhz
  Discrete Varying Lowpass3 : cstblocks/Linear Parameter Varying/Discrete Varying Lowpass  N=1  w0=0  Ts=Ts
      settings: SourceProductName=Control System Toolbox  SourceProductBaseCode=CT
  Gain2 : Gain  Gain=2*pi
  Product5 : Product
  Shapeit Integrator (Tustin) : Subsystem
  Shapeit Lead-Lag (Tustin) : Subsystem
  Out : Outport
  wires:
  Gain2/1 -> Discrete Varying Lowpass3/2
  Product5/1 -> Shapeit Integrator (Tustin)/1(In)
  Discrete Varying Lowpass3/1 -> Out/1
  Shapeit Integrator (Tustin)/1(Out) -> Shapeit Lead-Lag (Tustin)/1(In)
  Bus Selector/1 -> Product5/2  "<P_gain>"
  Bus Selector/2 -> Shapeit Integrator (Tustin)/2(I_fhz)  "<I_freq_hz>"
  param/1 -> Bus Selector/1
  Bus Selector/5 -> Gain2/1  "<LPF_fhz>"
  Bus Selector/4 -> Shapeit Lead-Lag (Tustin)/3(fp)  "<LL_pole_fhz>"
  reset_integrator/1 -> Shapeit Integrator (Tustin)/3(reset)
  Bus Selector/3 -> Shapeit Lead-Lag (Tustin)/2(fz)  "<LL_zero_fhz>"
  Shapeit Lead-Lag (Tustin)/1(Out) -> Discrete Varying Lowpass3/1
  In/1 -> Product5/1

== system ROPOD_4Wheel_TdistZMPC_cntr/Non-ROS Ropod Controller/platform vel cntr/Bumper Interaction Controller/Bumper_system/Lo-Pass filter1 ==
  s_data : Inport
  Constant : Constant  Value=2*pi*0.8
  Demux : Demux  Outputs=8
  Discrete Varying Lowpass{1..8} (8 alike) : cstblocks/Linear Parameter Varying/Discrete Varying Lowpass  N=1  w0=0  Ts=Ts
      settings: SourceProductName=Control System Toolbox  SourceProductBaseCode=CT
  LTI System{,1..7} (8 alike) : cstblocks/LTI System  Commented=through  sys=hpfD_Bumper  IC=[]
  Mux : Mux  Inputs=8
  Transfer Fcn1 : TransferFcn  Commented=on  Denominator=[(1/(2*pi*0.8)) 1]
  Transfer Fcn9 : TransferFcn  Commented=on  Numerator=[1 0 0]  Denominator=[1 (2*0.0003) 0.0003^2]
  Filterd_s_data : Outport
  wires:
  Mux/1 -> Filterd_s_data/1
  Discrete Varying Lowpass6/1 -> LTI System5/1
  Discrete Varying Lowpass5/1 -> LTI System4/1
  Discrete Varying Lowpass3/1 -> LTI System2/1
  Discrete Varying Lowpass1/1 -> LTI System1/1
  Discrete Varying Lowpass2/1 -> LTI System/1
  Demux/6 -> Discrete Varying Lowpass6/1
  Demux/5 -> Discrete Varying Lowpass5/1
  Demux/3 -> Discrete Varying Lowpass3/1
  Demux/2 -> Discrete Varying Lowpass1/1
  Demux/1 -> Discrete Varying Lowpass2/1
  s_data/1 -> Demux/1
  Demux/7 -> Discrete Varying Lowpass7/1
  Discrete Varying Lowpass7/1 -> LTI System6/1
  Demux/8 -> Discrete Varying Lowpass8/1
  Discrete Varying Lowpass8/1 -> LTI System7/1
  Demux/4 -> Discrete Varying Lowpass4/1
  Discrete Varying Lowpass4/1 -> LTI System3/1
  LTI System/1 -> Mux/1
  LTI System1/1 -> Mux/2
  LTI System2/1 -> Mux/3
  LTI System3/1 -> Mux/4
  LTI System4/1 -> Mux/5
  LTI System5/1 -> Mux/6
  LTI System6/1 -> Mux/7
  LTI System7/1 -> Mux/8
  Constant/1 -> Discrete Varying Lowpass8/2, Discrete Varying Lowpass7/2, Discrete Varying Lowpass6/2, Discrete Varying Lowpass5/2, Discrete Varying Lowpass4/2, Discrete Varying Lowpass3/2, Discrete Varying Lowpass1/2, Discrete Varying Lowpass2/2

== system ROPOD_4Wheel_TdistZMPC_cntr/Non-ROS Ropod Controller/platform vel cntr/Bumper Interaction Controller/Bumper_system/Lo-Pass filter2 ==
  s_data : Inport
  Constant : Constant  Value=2*pi*0.8
  Demux : Demux  Outputs=8
  Discrete Varying Lowpass{1..8} (8 alike) : cstblocks/Linear Parameter Varying/Discrete Varying Lowpass  N=1  w0=0  Ts=Ts
      settings: SourceProductName=Control System Toolbox  SourceProductBaseCode=CT
  LTI System{,1..7} (8 alike) : cstblocks/LTI System  Commented=through  sys=hpfD_Bumper  IC=[]
  Mux : Mux  Inputs=8
  Transfer Fcn1 : TransferFcn  Commented=on  Denominator=[(1/(2*pi*0.8)) 1]
  Transfer Fcn9 : TransferFcn  Commented=on  Numerator=[1 0 0]  Denominator=[1 (2*0.0003) 0.0003^2]
  Filterd_s_data : Outport
  wires:
  Mux/1 -> Filterd_s_data/1
  Discrete Varying Lowpass6/1 -> LTI System5/1
  Discrete Varying Lowpass5/1 -> LTI System4/1
  Discrete Varying Lowpass3/1 -> LTI System2/1
  Discrete Varying Lowpass1/1 -> LTI System1/1
  Discrete Varying Lowpass2/1 -> LTI System/1
  Demux/6 -> Discrete Varying Lowpass6/1
  Demux/5 -> Discrete Varying Lowpass5/1
  Demux/3 -> Discrete Varying Lowpass3/1
  Demux/2 -> Discrete Varying Lowpass1/1
  Demux/1 -> Discrete Varying Lowpass2/1
  s_data/1 -> Demux/1
  Demux/7 -> Discrete Varying Lowpass7/1
  Discrete Varying Lowpass7/1 -> LTI System6/1
  Demux/8 -> Discrete Varying Lowpass8/1
  Discrete Varying Lowpass8/1 -> LTI System7/1
  Demux/4 -> Discrete Varying Lowpass4/1
  Discrete Varying Lowpass4/1 -> LTI System3/1
  LTI System/1 -> Mux/1
  LTI System1/1 -> Mux/2
  LTI System2/1 -> Mux/3
  LTI System3/1 -> Mux/4
  LTI System4/1 -> Mux/5
  LTI System5/1 -> Mux/6
  LTI System6/1 -> Mux/7
  LTI System7/1 -> Mux/8
  Constant/1 -> Discrete Varying Lowpass8/2, Discrete Varying Lowpass7/2, Discrete Varying Lowpass6/2, Discrete Varying Lowpass5/2, Discrete Varying Lowpass4/2, Discrete Varying Lowpass3/2, Discrete Varying Lowpass1/2, Discrete Varying Lowpass2/2

== system ROPOD_4Wheel_TdistZMPC_cntr/Non-ROS Ropod Controller/platform vel cntr/Bumper Interaction Controller/Bumper_system/Lo-Pass filter3 ==
  s_data : Inport
  Constant : Constant  Value=2*pi*0.8
  Demux : Demux  Outputs=8
  Discrete Varying Lowpass{1..8} (8 alike) : cstblocks/Linear Parameter Varying/Discrete Varying Lowpass  N=1  w0=0  Ts=Ts
      settings: SourceProductName=Control System Toolbox  SourceProductBaseCode=CT
  LTI System{,1..7} (8 alike) : cstblocks/LTI System  Commented=through  sys=hpfD_Bumper  IC=[]
  Mux : Mux  Inputs=8
  Transfer Fcn1 : TransferFcn  Commented=on  Denominator=[(1/(2*pi*0.8)) 1]
  Transfer Fcn9 : TransferFcn  Commented=on  Numerator=[1 0 0]  Denominator=[1 (2*0.0003) 0.0003^2]
  Filterd_s_data : Outport
  wires:
  Mux/1 -> Filterd_s_data/1
  Discrete Varying Lowpass6/1 -> LTI System5/1
  Discrete Varying Lowpass5/1 -> LTI System4/1
  Discrete Varying Lowpass3/1 -> LTI System2/1
  Discrete Varying Lowpass1/1 -> LTI System1/1
  Discrete Varying Lowpass2/1 -> LTI System/1
  Demux/6 -> Discrete Varying Lowpass6/1
  Demux/5 -> Discrete Varying Lowpass5/1
  Demux/3 -> Discrete Varying Lowpass3/1
  Demux/2 -> Discrete Varying Lowpass1/1
  Demux/1 -> Discrete Varying Lowpass2/1
  s_data/1 -> Demux/1
  Demux/7 -> Discrete Varying Lowpass7/1
  Discrete Varying Lowpass7/1 -> LTI System6/1
  Demux/8 -> Discrete Varying Lowpass8/1
  Discrete Varying Lowpass8/1 -> LTI System7/1
  Demux/4 -> Discrete Varying Lowpass4/1
  Discrete Varying Lowpass4/1 -> LTI System3/1
  LTI System/1 -> Mux/1
  LTI System1/1 -> Mux/2
  LTI System2/1 -> Mux/3
  LTI System3/1 -> Mux/4
  LTI System4/1 -> Mux/5
  LTI System5/1 -> Mux/6
  LTI System6/1 -> Mux/7
  LTI System7/1 -> Mux/8
  Constant/1 -> Discrete Varying Lowpass8/2, Discrete Varying Lowpass7/2, Discrete Varying Lowpass6/2, Discrete Varying Lowpass5/2, Discrete Varying Lowpass4/2, Discrete Varying Lowpass3/2, Discrete Varying Lowpass1/2, Discrete Varying Lowpass2/2

== system ROPOD_4Wheel_TdistZMPC_cntr/Non-ROS Ropod Controller/platform vel cntr/Bumper Interaction Controller/Bumper_system/Lo-Pass filter4 ==
  s_data : Inport
  Constant : Constant  Value=2*pi*0.8
  Demux : Demux  Outputs=8
  Discrete Varying Lowpass{1..8} (8 alike) : cstblocks/Linear Parameter Varying/Discrete Varying Lowpass  N=1  w0=0  Ts=Ts
      settings: SourceProductName=Control System Toolbox  SourceProductBaseCode=CT
  LTI System{,1..7} (8 alike) : cstblocks/LTI System  Commented=through  sys=hpfD_Bumper  IC=[]
  Mux : Mux  Inputs=8
  Transfer Fcn1 : TransferFcn  Commented=on  Denominator=[(1/(2*pi*0.8)) 1]
  Transfer Fcn9 : TransferFcn  Commented=on  Numerator=[1 0 0]  Denominator=[1 (2*0.0003) 0.0003^2]
  Filterd_s_data : Outport
  wires:
  Mux/1 -> Filterd_s_data/1
  Discrete Varying Lowpass6/1 -> LTI System5/1
  Discrete Varying Lowpass5/1 -> LTI System4/1
  Discrete Varying Lowpass3/1 -> LTI System2/1
  Discrete Varying Lowpass1/1 -> LTI System1/1
  Discrete Varying Lowpass2/1 -> LTI System/1
  Demux/6 -> Discrete Varying Lowpass6/1
  Demux/5 -> Discrete Varying Lowpass5/1
  Demux/3 -> Discrete Varying Lowpass3/1
  Demux/2 -> Discrete Varying Lowpass1/1
  Demux/1 -> Discrete Varying Lowpass2/1
  s_data/1 -> Demux/1
  Demux/7 -> Discrete Varying Lowpass7/1
  Discrete Varying Lowpass7/1 -> LTI System6/1
  Demux/8 -> Discrete Varying Lowpass8/1
  Discrete Varying Lowpass8/1 -> LTI System7/1
  Demux/4 -> Discrete Varying Lowpass4/1
  Discrete Varying Lowpass4/1 -> LTI System3/1
  LTI System/1 -> Mux/1
  LTI System1/1 -> Mux/2
  LTI System2/1 -> Mux/3
  LTI System3/1 -> Mux/4
  LTI System4/1 -> Mux/5
  LTI System5/1 -> Mux/6
  LTI System6/1 -> Mux/7
  LTI System7/1 -> Mux/8
  Constant/1 -> Discrete Varying Lowpass8/2, Discrete Varying Lowpass7/2, Discrete Varying Lowpass6/2, Discrete Varying Lowpass5/2, Discrete Varying Lowpass4/2, Discrete Varying Lowpass3/2, Discrete Varying Lowpass1/2, Discrete Varying Lowpass2/2

== system ROPOD_4Wheel_TdistZMPC_cntr/Non-ROS Ropod Controller/platform vel cntr/Bumper Interaction Controller/Bumper_system/cal ==
  In1 : Inport
  Calibration1 : MATLAB Function  TreatAsAtomicUnit=on
  Memory2 : Memory  InitialCondition=1
  Memory3 : Memory
  Out1 : Outport
  wires:
  Calibration1/2(i) -> Memory2/1
  Memory2/1 -> Calibration1/2(sample)
  Memory3/1 -> Calibration1/3(data)
  In1/1 -> Calibration1/1(angle)
  Calibration1/1(cal_angle) -> Out1/1
  Calibration1/3(data_out) -> Memory3/1

== system ROPOD_4Wheel_TdistZMPC_cntr/Non-ROS Ropod Controller/platform vel cntr/Bumper Interaction Controller/Bumper_system/cal1 ==
  In1 : Inport
  Calibration1 : MATLAB Function  TreatAsAtomicUnit=on
  Memory2 : Memory  InitialCondition=1
  Memory3 : Memory
  Out1 : Outport
  wires:
  Calibration1/3(data_out) -> Memory3/1
  Calibration1/1(cal_angle) -> Out1/1
  In1/1 -> Calibration1/1(angle)
  Memory3/1 -> Calibration1/3(data)
  Memory2/1 -> Calibration1/2(sample)
  Calibration1/2(i) -> Memory2/1
